simulink model "FINITE_TIME_CONVERGENCE"  (R2020b)
settings: Solver=FixedStepAuto  StartTime=0.0  StopTime=40  FixedStep=0.001  RelTol=1e-7
settings Model: Creator=cyx  LastModifiedBy=cyx
settings SolverCC: ZeroCrossAlgorithm=Adaptive  AlgebraicLoopSolver=LineSearch
settings DataIOCC: ReturnWorkspaceOutputs=off

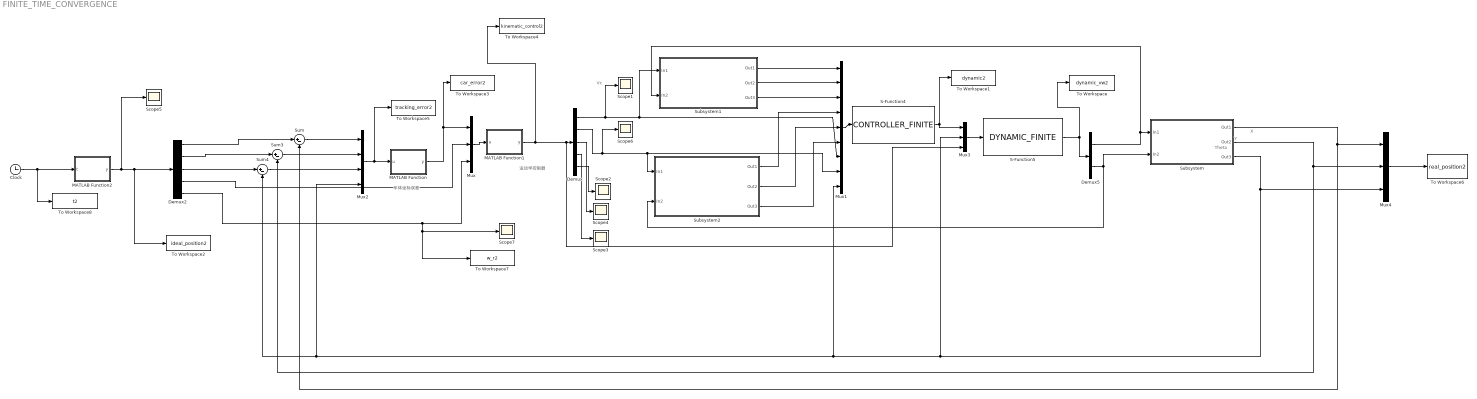
== system FINITE_TIME_CONVERGENCE ==
  note: Theta
  note: X
  note: 运动学控制器
  note: Vc
  note: Y
  note: 车体坐标误差
  Clock : Clock
  Demux : Demux  Outputs=5
  Demux2 : Demux  Outputs=5
  Demux5 : Demux  Outputs=2
  MATLAB Function : MATLAB Function  TreatAsAtomicUnit=on
  MATLAB Function1 : MATLAB Function  TreatAsAtomicUnit=on
  MATLAB Function2 : MATLAB Function  TreatAsAtomicUnit=on
  Mux : Mux  Inputs=3
  Mux1 : Mux  Inputs=[1 1 1 1 1 1 1 1 1]
  Mux2 : Mux
  Mux3 : Mux  Inputs=3
  Mux4 : Mux  Inputs=3
  S-Function4 : S-Function  FunctionName=CONTROLLER_FINITE  SFunctionDeploymentMode=off  EnableBusSupport=off
  S-Function5 : S-Function  FunctionName=DYNAMIC_FINITE  SFunctionDeploymentMode=off  EnableBusSupport=off
  Scope{1..7} (7 alike) : Scope
  Subsystem : Subsystem
  Subsystem1 : Subsystem
  Subsystem2 : Subsystem
  Sum : Sum  Inputs=|+-
  Sum3 : Sum  Inputs=|+-
  Sum4 : Sum  Inputs=|+-
  To Workspace : ToWorkspace  VariableName=dynamic_vw2  SampleTime=-1
  To Workspace1 : ToWorkspace  VariableName=dynamic2  SampleTime=-1
  To Workspace2 : ToWorkspace  VariableName=ideal_position2  SampleTime=-1
  To Workspace3 : ToWorkspace  VariableName=car_error2  SampleTime=-1
  To Workspace4 : ToWorkspace  VariableName=kinematic_control2  SampleTime=-1
  To Workspace5 : ToWorkspace  VariableName=tracking_error2  SampleTime=-1
  To Workspace6 : ToWorkspace  VariableName=real_position2  SampleTime=-1
      settings: Save2DSignal=2-D array (concatenate along first dimension)
  To Workspace7 : ToWorkspace  VariableName=w_r2  SampleTime=-1
  To Workspace8 : ToWorkspace  VariableName=t2  SampleTime=-1
  wires:
  Sum3/1 -> Mux2/2
  Subsystem1/3(Out3) -> Mux1/3
  Demux5/1 -> Subsystem1/2(In2), Subsystem/1(In1)
  Subsystem2/3(Out3) -> Mux1/6
  Demux/5 -> Scope2/1
  MATLAB Function1/1(y) -> Mux3/3, Demux/1, To Workspace4/1
  Subsystem1/2(Out2) -> Mux1/2
  Sum/1 -> Mux2/1
  Subsystem1/1(Out1) -> Mux1/1
  MATLAB Function/1(y) -> To Workspace3/1, Mux/1
  Subsystem/1(Out1) -> Mux4/1, Sum/2
  Mux4/1 -> To Workspace6/1
  Demux/1 -> Scope1/1, Subsystem1/1(In1), Mux1/7
  Subsystem2/1(Out1) -> Mux1/4
  S-Function5/1 -> Demux5/1, To Workspace/1
  Demux2/4 -> Mux/2
  Mux3/1 -> S-Function5/1
  S-Function4/1 -> To Workspace1/1, Mux3/1
  Demux2/3 -> Sum4/1
  Mux2/1 -> To Workspace5/1, MATLAB Function/1(u)
  Demux5/2 -> Subsystem/2(In2), Subsystem2/2(In2)
  Clock/1 -> To Workspace8/1, MATLAB Function2/1(t)
  Subsystem/2(Out2) -> Sum3/2, Mux4/2
  Sum4/1 -> Mux2/3
  Subsystem/3(Out3) -> Mux2/4, Sum4/2, Mux1/9, Mux3/2, Mux4/3
  Mux/1 -> MATLAB Function1/1(u)
  Demux2/2 -> Sum3/1
  Mux1/1 -> S-Function4/1
  Demux/2 -> Scope6/1, Subsystem2/1(In1), Mux1/8
  MATLAB Function2/1(y) -> Scope5/1, To Workspace2/1, Demux2/1
  Subsystem2/2(Out2) -> Mux1/5
  Demux/3 -> Scope4/1
  Demux/4 -> Scope3/1
  Demux2/1 -> Sum/1
  Demux2/5 -> To Workspace7/1, Scope7/1, Mux/3

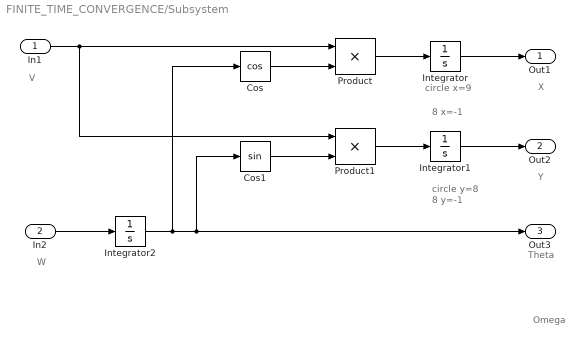
== system FINITE_TIME_CONVERGENCE/Subsystem ==
  note: circle x=9
  note: W
  note: V
  note: X
  note: Y
  note: Theta
  note: Omega
  note: circle y=8
  note: 8 x=-1
  note: 8 y=-1
  In1 : Inport
  In2 : Inport  Port=2
  Cos : Trigonometry  Operator=cos
  Cos1 : Trigonometry
  Integrator : Integrator  InitialCondition=4
  Integrator1 : Integrator  InitialCondition=4
  Integrator2 : Integrator
  Product : Product
  Product1 : Product
  Out1 : Outport
  Out2 : Outport  Port=2
  Out3 : Outport  Port=3
  wires:
  In1/1 -> Product1/1, Product/1
  Product/1 -> Integrator/1
  Integrator/1 -> Out1/1
  Cos/1 -> Product/2
  Integrator1/1 -> Out2/1
  In2/1 -> Integrator2/1
  Integrator2/1 -> Cos1/1, Out3/1, Cos/1
  Product1/1 -> Integrator1/1
  Cos1/1 -> Product1/2

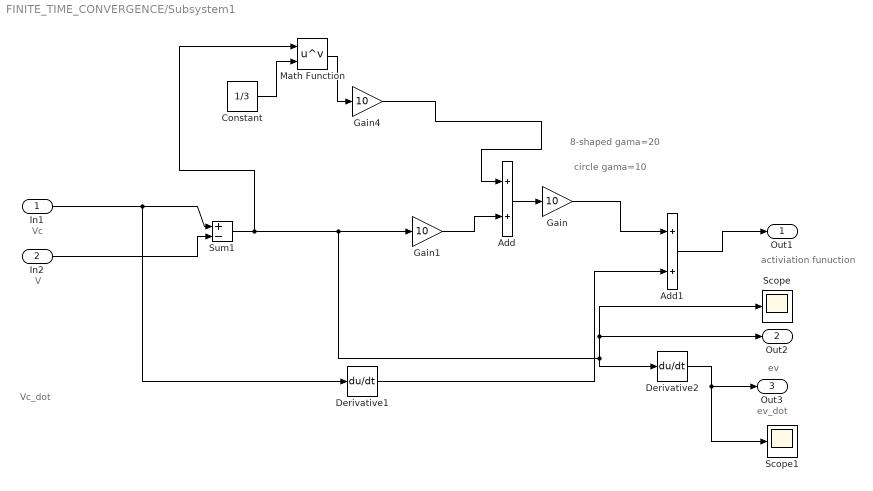
== system FINITE_TIME_CONVERGENCE/Subsystem1 ==
  note: 8-shaped gama=20
  note: Vc
  note: V
  note: Vc_dot
  note: ev_dot
  note: activiation funuction
  note: ev
  note: circle gama=10
  In1 : Inport
  In2 : Inport  Port=2
  Add : Sum
  Add1 : Sum
  Constant : Constant  Value=1/3
  Derivative1 : Derivative
  Derivative2 : Derivative
  Gain : Gain  Gain=10
  Gain1 : Gain  Gain=10
  Gain4 : Gain  Gain=10
  Math Function : Math  Operator=pow  SignedPower=on  SaturateOnIntegerOverflow=on
  Scope : Scope
  Scope1 : Scope
  Sum1 : Sum  Inputs=|+-
  Out1 : Outport
  Out2 : Outport  Port=2
  Out3 : Outport  Port=3
  wires:
  Derivative2/1 -> Scope1/1, Out3/1
  In1/1 -> Derivative1/1, Sum1/1
  In2/1 -> Sum1/2
  Add/1 -> Gain/1
  Gain/1 -> Add1/1
  Add1/1 -> Out1/1
  Derivative1/1 -> Add1/2
  Gain1/1 -> Add/2
  Gain4/1 -> Add/1
  Sum1/1 -> Math Function/1, Scope/1, Out2/1, Derivative2/1, Gain1/1
  Math Function/1 -> Gain4/1
  Constant/1 -> Math Function/2

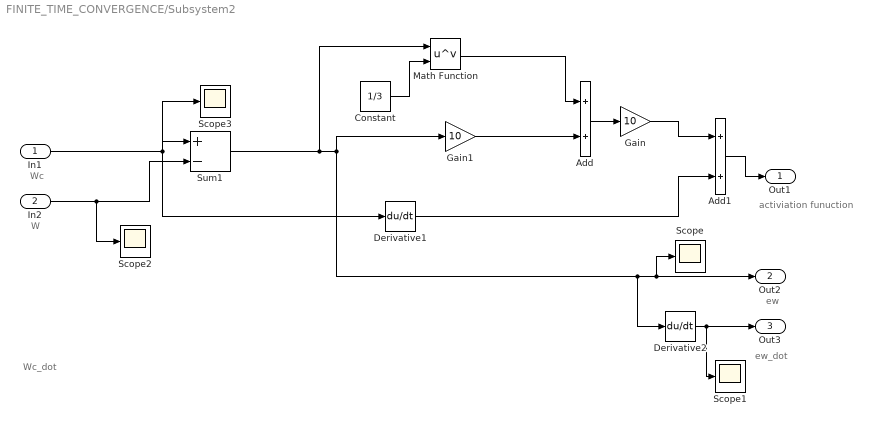
== system FINITE_TIME_CONVERGENCE/Subsystem2 ==
  note: Wc
  note: W
  note: Wc_dot
  note: ew_dot
  note: activiation funuction
  note: ew
  In1 : Inport
  In2 : Inport  Port=2
  Add : Sum
  Add1 : Sum
  Constant : Constant  Value=1/3
  Derivative1 : Derivative
  Derivative2 : Derivative
  Gain : Gain  Gain=10
  Gain1 : Gain  Gain=10
  Math Function : Math  Operator=pow  SignedPower=on  SaturateOnIntegerOverflow=on
  Scope{,1..3} (4 alike) : Scope
  Sum1 : Sum  Inputs=|+-
  Out1 : Outport
  Out2 : Outport  Port=2
  Out3 : Outport  Port=3
  wires:
  Derivative2/1 -> Scope1/1, Out3/1
  In1/1 -> Derivative1/1, Sum1/1, Scope3/1
  In2/1 -> Scope2/1, Sum1/2
  Add/1 -> Gain/1
  Gain/1 -> Add1/1
  Add1/1 -> Out1/1
  Derivative1/1 -> Add1/2
  Gain1/1 -> Add/2
  Constant/1 -> Math Function/2
  Sum1/1 -> Math Function/1, Derivative2/1, Scope/1, Out2/1, Gain1/1
  Math Function/1 -> Add/1

== matlab function FINITE_TIME_CONVERGENCE/MATLAB Function ==
  data: u input; y output
function y = fcn(u)
%%讲机器人误差坐标进行转换；
%转换矩阵C

C=[cos(u(4))   sin(u(4))      0;
    -sin(u(4)) cos(u(4))    0;
    0            0          1];

%%将世界坐标系下的误差转化至车体坐标下转换后的误差q_e=[e1 e2 e3]
%输入为世界坐标系下的误差x_e,y_e,theta_e对应u(1),u(2)
e1=C(1,1)*u(1)+C(1,2)*u(2);
e2=C(2,1)*u(1)+C(2,2)*u(2);
e3=C(3,3)*u(3);
y =[e1;e2;e3];

== matlab function FINITE_TIME_CONVERGENCE/MATLAB Function2 ==
  data: t input; y output
function y = input(t)

S=1;
switch S
    case 1%圆形轨迹
       w_r=1;
       x_r= 5*cos(w_r*t);
       y_r= 5+5*sin(w_r*t);
       theta_r=w_r*t;
        v_r=5;
       %theta_r=atan2(x_r,y_r);
        
    case 2 %8轨迹
        x_r=10*sin(t/10);
        y_r=10*sin(t/20);
        dx_r=cos(t/10);
        dy_r=0.5*cos(t/20);
        v_r=sqrt(dy_r.^2+dx_r.^2);
        if atan2(dy_r,dx_r)>0
            theta_r=atan2(dy_r,dx_r);
        else
            theta_r=atan2(dy_r,dx_r)+2*pi;
        end
        w_r=0.5;
   
    case 3 %圆角矩形
        x_r=sign(cos(t)).*sqrt(abs(100*cos(t)));
        y_r=sign(sin(t)).*sqrt(abs(100*sin(t)));
        theta_r=atan2(y_r,x_r);
        if 0<t && t<3.146 | 10<t && t<13.146 | 20<t && t<23.146 | 30<t && t<33.146
            v_r=1;
            w_r=0.5;
        else
            v_r=1;
            w_r=0;
        end
 
end


y =[x_r; y_r; theta_r; v_r; w_r];

== matlab function FINITE_TIME_CONVERGENCE/MATLAB Function1 ==
  data: u input; y output
function y = kinematic_controller(u)

%e1=u(1);
%e2=u(2);
%e3=u(3);

ex=u(1);
ey=u(2);
etheta=u(3);

v_r=u(4);
w_r=u(5);

%%机器人反演控制律；控制输入为参考速度v_r,w_r以及三个车体坐标系误差；

%---------有限时间控制律-----
%k1=6;k2=2;k3=2;
%v_c=v_r+k2*sqrt(abs(e1))*sign(e1)-k3*w_r*sqrt(abs(e2))*sign(e2);
%w_c=w_r+k1*sqrt(abs(e3))*sign(e3);


%--------反步法控制律---------
%k1=100;k2=50;k3=5;
%v_c=v_r*cos(e3)+k1*e1;
%w_c=w_r+k2*v_r*e2+k3*v_r*sin(e3);

%--------控制律2
%v_c=v_r*cos(e3)+k1*e1;
%w_c=w_r+k2*v_r*e2+k3*v_r*sin(e3);

%----------------反演法控制率u--------------
k1=0.1;k2=50;k3=150;k4=10;
w_c=2*k3*ey*v_r*cos(etheta/2)+k4*sin(etheta/2)+w_r;
vrdot=0;
wrdot=0;
omega_dot=2*k3*((-w_c*ex+v_r*sin(etheta))*v_r+ey*vrdot)*cos(etheta/2)-k3*ey*v_r*sin(etheta/2)*(w_r-w_c)...
    +0.5*k4*cos(etheta/2)*(w_r-w_c)+wrdot;
v_c=v_r*cos(etheta)+k1*w_c*ex*(w_c/(1+w_c^2)^0.5)-k1*v_r*sin(etheta)*(w_c/(1+w_c^2)^0.5)...
    -k1*omega_dot*ey/(1+w_c^2)^1.5+k2*(ex-k1*ey*(w_c/(1+w_c^2)^0.5))-0.06;



%------------------FCZNN控制率u-------------------
%gama=10;k=20;
%phi1=power(ex,3)+k*ex+nthroot(ex,3); 
%phi2=power(ey,3)+k*ey+nthroot(ey,3);
%phi3=power(etheta,3)+k*etheta+nthroot(etheta,3);
%v_c=ey*((w_r+gama*phi3+v_r*sin(etheta)+gama*phi2)/(ex+1))+v_r*cos(etheta)+gama*phi1;
%w_c=((w_r+gama*phi3+v_r*sin(etheta)+gama*phi2)/(ex+1));%w

%限制输出-----------
if abs(v_c)>6
    v_c=sign(v_c)*6;
end
if abs(w_c)>6
    w_c=sign(w_c)*6;
end


e1_dot=w_c*ey-v_c+v_r*cos(etheta);
e2_dot=-w_c*ex+v_r*sin(etheta);
e3_dot=w_r-w_c;

y = [v_c;w_c;e1_dot;e2_dot;e3_dot];
